simulink library "Computer_Library"  (Simulink 8.1)
settings: Solver=ode45  StartTime=0.0  StopTime=10.0  RelTol=1e-3
values from neighbouring files (symbols this model uses):
  A = 10    [CharTable.m]
  ARROW_DOWN = 48    [CharTable.m]
  ARROW_LEFT = 49    [CharTable.m]
  ARROW_RIGHT = 50    [CharTable.m]
  ARROW_UP = 47    [CharTable.m]
  ASTERISK = 39    [CharTable.m]
  B = 11    [CharTable.m]
  BACKSLASH = 43    [CharTable.m]
  C = 12    [CharTable.m]
  COLON = 40    [CharTable.m]
  COMMA = 53    [CharTable.m]
  CROSS = 38    [CharTable.m]
  CURSOR = 62    [CharTable.m]
  D = 13    [CharTable.m]
  DOT = 52    [CharTable.m]
  EQUAL = 44    [CharTable.m]
  EXCLAMATION_MARK = 55    [CharTable.m]
  F = 15    [CharTable.m]
  G = 16    [CharTable.m]
  GREATER_THAN = 46    [CharTable.m]
  H = 17    [CharTable.m]
  I = 18    [CharTable.m]
  J = 19    [CharTable.m]
  K = 20    [CharTable.m]
  L = 21    [CharTable.m]
  LEFT_PARENTHESES = 59    [CharTable.m]
  LESS_THAN = 45    [CharTable.m]
  M = 22    [CharTable.m]
  MINUS = 37    [CharTable.m]
  N = 23    [CharTable.m]
  O = 24    [CharTable.m]
  P = 25    [CharTable.m]
  PERCENT = 58    [CharTable.m]
  PLUS = 36    [CharTable.m]
  Q = 32    [CharTable.m]
  QUESTION_MARK = 54    [CharTable.m]
  QUOTE = 56    [CharTable.m]
  R = 26    [CharTable.m]
  RECTANGLE = 63    [CharTable.m]
  RIGHT_PARENTHESES = 60    [CharTable.m]
  RomCode = reshape(transpose(RomCode), [], 1)    [ROM.m]
  S = 27    [CharTable.m]
  SEMICOLON = 41    [CharTable.m]
  SHARP = 57    [CharTable.m]
  SLASH = 42    [CharTable.m]
  SPACE = 61    [CharTable.m]
  T = 28    [CharTable.m]
  U = 29    [CharTable.m]
  UNDERSCORE = 51    [CharTable.m]
  V = 30    [CharTable.m]
  W = 31    [CharTable.m]
  X = 33    [CharTable.m]
  Y = 34    [CharTable.m]
  Z = 35    [CharTable.m]
undefined symbols (not defined in the file or in its folder): char_0
libraries: Memory_Blocks_Lib x116, Byte_Multiplexers_Lib x44, commutil2 x18, Bit_Multiplexers_Lib x17, Decoders_Lib x9, simulink_extras x8, Logic_Operations_Lib x4, Byte_Demultiplexers_Lib x2, Arithmetic_Operations_Lib x2, dspsnks4 x1
(part 2 of 4)

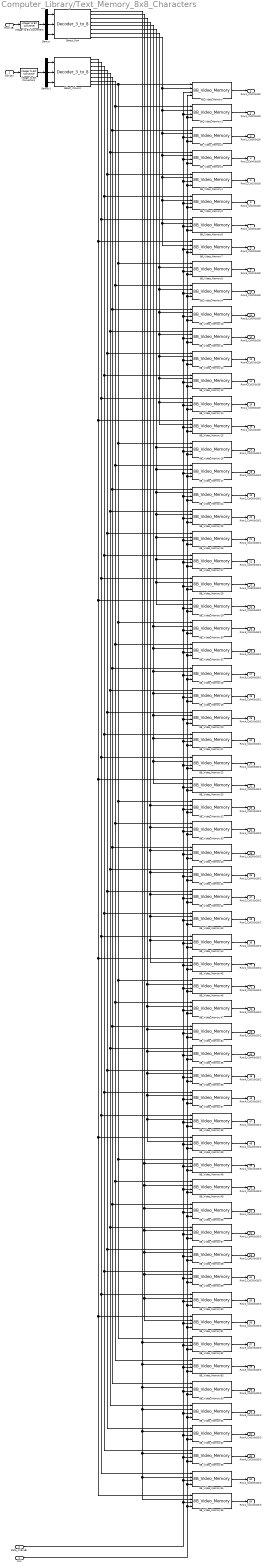
== system Computer_Library/Text_Memory_8x8_Characters ==
  Row(1B) : Inport
  Col(1B) : Inport  Port=2
  Data_In(8x1B) : Inport  Port=3
  CLK : Inport  Port=4
  8B_Video_Memory{,1..63} (64 alike) : Memory_Blocks_Lib/Memory_Blocks_Lib/8B_Video_Memory
  Demux : Demux  Outputs=3
  Demux1 : Demux  Outputs=3
  Integer to Bit Converter3 : commutil2/Integer to Bit Converter  nbits=3  signedInputValues=Unsigned  bitOrder=MSB first  outDtype=uint8
  Integer to Bit Converter4 : commutil2/Integer to Bit Converter  nbits=3  signedInputValues=Unsigned  bitOrder=MSB first  outDtype=uint8
  Select_Column : Decoders_Lib/Decoders_Lib/Decoder_3_to_8
  Select_Row : Decoders_Lib/Decoders_Lib/Decoder_3_to_8
  Row1_Col1(8x1B) : Outport
  Row1_Col2(8x1B) : Outport  Port=2
  Row1_Col3(8x1B) : Outport  Port=3
  Row1_Col4(8x1B) : Outport  Port=4
  Row2_Col1(8x1B) : Outport  Port=5
  Row2_Col2(8x1B) : Outport  Port=6
  Row2_Col3(8x1B) : Outport  Port=7
  Row2_Col4(8x1B) : Outport  Port=8
  Row3_Col1(8x1B) : Outport  Port=9
  Row3_Col2(8x1B) : Outport  Port=10
  Row3_Col3(8x1B) : Outport  Port=11
  Row3_Col4(8x1B) : Outport  Port=12
  Row4_Col1(8x1B) : Outport  Port=13
  Row4_Col2(8x1B) : Outport  Port=14
  Row4_Col3(8x1B) : Outport  Port=15
  Row4_Col4(8x1B) : Outport  Port=16
  Row1_Col1(8x1B)1 : Outport  Port=17
  Row1_Col2(8x1B)1 : Outport  Port=18
  Row1_Col3(8x1B)1 : Outport  Port=19
  Row1_Col4(8x1B)1 : Outport  Port=20
  Row2_Col1(8x1B)1 : Outport  Port=21
  Row2_Col2(8x1B)1 : Outport  Port=22
  Row2_Col3(8x1B)1 : Outport  Port=23
  Row2_Col4(8x1B)1 : Outport  Port=24
  Row3_Col1(8x1B)1 : Outport  Port=25
  Row3_Col2(8x1B)1 : Outport  Port=26
  Row3_Col3(8x1B)1 : Outport  Port=27
  Row3_Col4(8x1B)1 : Outport  Port=28
  Row4_Col1(8x1B)1 : Outport  Port=29
  Row4_Col2(8x1B)1 : Outport  Port=30
  Row4_Col3(8x1B)1 : Outport  Port=31
  Row4_Col4(8x1B)1 : Outport  Port=32
  Row1_Col1(8x1B)2 : Outport  Port=33
  Row1_Col2(8x1B)2 : Outport  Port=34
  Row1_Col3(8x1B)2 : Outport  Port=35
  Row1_Col4(8x1B)2 : Outport  Port=36
  Row2_Col1(8x1B)2 : Outport  Port=37
  Row2_Col2(8x1B)2 : Outport  Port=38
  Row2_Col3(8x1B)2 : Outport  Port=39
  Row2_Col4(8x1B)2 : Outport  Port=40
  Row3_Col1(8x1B)2 : Outport  Port=41
  Row3_Col2(8x1B)2 : Outport  Port=42
  Row3_Col3(8x1B)2 : Outport  Port=43
  Row3_Col4(8x1B)2 : Outport  Port=44
  Row4_Col1(8x1B)2 : Outport  Port=45
  Row4_Col2(8x1B)2 : Outport  Port=46
  Row4_Col3(8x1B)2 : Outport  Port=47
  Row4_Col4(8x1B)2 : Outport  Port=48
  Row1_Col1(8x1B)3 : Outport  Port=49
  Row1_Col2(8x1B)3 : Outport  Port=50
  Row1_Col3(8x1B)3 : Outport  Port=51
  Row1_Col4(8x1B)3 : Outport  Port=52
  Row2_Col1(8x1B)3 : Outport  Port=53
  Row2_Col2(8x1B)3 : Outport  Port=54
  Row2_Col3(8x1B)3 : Outport  Port=55
  Row2_Col4(8x1B)3 : Outport  Port=56
  Row3_Col1(8x1B)3 : Outport  Port=57
  Row3_Col2(8x1B)3 : Outport  Port=58
  Row3_Col3(8x1B)3 : Outport  Port=59
  Row3_Col4(8x1B)3 : Outport  Port=60
  Row4_Col1(8x1B)3 : Outport  Port=61
  Row4_Col2(8x1B)3 : Outport  Port=62
  Row4_Col3(8x1B)3 : Outport  Port=63
  Row4_Col4(8x1B)3 : Outport  Port=64
  wires:
  Row(1B)/1 -> Integer to Bit Converter3/1
  Integer to Bit Converter3/1 -> Demux/1
  Col(1B)/1 -> Integer to Bit Converter4/1
  Integer to Bit Converter4/1 -> Demux1/1
  8B_Video_Memory/1 -> Row1_Col1(8x1B)/1
  8B_Video_Memory1/1 -> Row1_Col2(8x1B)/1
  8B_Video_Memory2/1 -> Row1_Col3(8x1B)/1
  8B_Video_Memory3/1 -> Row1_Col4(8x1B)/1
  Select_Row/5 -> 8B_Video_Memory30/2, 8B_Video_Memory31/2, 8B_Video_Memory18/2, 8B_Video_Memory19/2, 8B_Video_Memory20/2, 8B_Video_Memory21/2, 8B_Video_Memory22/2, 8B_Video_Memory23/2
  Select_Row/6 -> 8B_Video_Memory16/2, 8B_Video_Memory17/2, 8B_Video_Memory24/2, 8B_Video_Memory25/2, 8B_Video_Memory26/2, 8B_Video_Memory27/2, 8B_Video_Memory28/2, 8B_Video_Memory29/2
  Select_Column/5 -> 8B_Video_Memory3/1, 8B_Video_Memory51/1, 8B_Video_Memory57/1, 8B_Video_Memory35/1, 8B_Video_Memory41/1, 8B_Video_Memory19/1, 8B_Video_Memory25/1, 8B_Video_Memory11/1
  Select_Column/6 -> 8B_Video_Memory2/1, 8B_Video_Memory50/1, 8B_Video_Memory56/1, 8B_Video_Memory34/1, 8B_Video_Memory40/1, 8B_Video_Memory18/1, 8B_Video_Memory24/1, 8B_Video_Memory10/1
  Select_Row/8 -> 8B_Video_Memory/2, 8B_Video_Memory1/2, 8B_Video_Memory2/2, 8B_Video_Memory3/2, 8B_Video_Memory4/2, 8B_Video_Memory5/2, 8B_Video_Memory6/2, 8B_Video_Memory7/2
  Select_Row/7 -> 8B_Video_Memory8/2, 8B_Video_Memory9/2, 8B_Video_Memory10/2, 8B_Video_Memory11/2, 8B_Video_Memory12/2, 8B_Video_Memory13/2, 8B_Video_Memory14/2, 8B_Video_Memory15/2
  Select_Column/8 -> 8B_Video_Memory/1, 8B_Video_Memory62/1, 8B_Video_Memory48/1, 8B_Video_Memory46/1, 8B_Video_Memory32/1, 8B_Video_Memory30/1, 8B_Video_Memory16/1, 8B_Video_Memory8/1
  Select_Column/7 -> 8B_Video_Memory1/1, 8B_Video_Memory63/1, 8B_Video_Memory49/1, 8B_Video_Memory47/1, 8B_Video_Memory33/1, 8B_Video_Memory31/1, 8B_Video_Memory17/1, 8B_Video_Memory9/1
  8B_Video_Memory4/1 -> Row2_Col1(8x1B)/1
  8B_Video_Memory5/1 -> Row2_Col2(8x1B)/1
  8B_Video_Memory6/1 -> Row2_Col3(8x1B)/1
  8B_Video_Memory7/1 -> Row2_Col4(8x1B)/1
  8B_Video_Memory8/1 -> Row3_Col1(8x1B)/1
  8B_Video_Memory9/1 -> Row3_Col2(8x1B)/1
  8B_Video_Memory10/1 -> Row3_Col3(8x1B)/1
  8B_Video_Memory11/1 -> Row3_Col4(8x1B)/1
  8B_Video_Memory12/1 -> Row4_Col1(8x1B)/1
  8B_Video_Memory13/1 -> Row4_Col2(8x1B)/1
  8B_Video_Memory14/1 -> Row4_Col3(8x1B)/1
  8B_Video_Memory15/1 -> Row4_Col4(8x1B)/1
  Demux/1 -> Select_Row/1
  Demux/2 -> Select_Row/2
  Demux1/1 -> Select_Column/1
  Demux1/2 -> Select_Column/2
  8B_Video_Memory16/1 -> Row1_Col1(8x1B)1/1
  8B_Video_Memory17/1 -> Row1_Col2(8x1B)1/1
  8B_Video_Memory24/1 -> Row1_Col3(8x1B)1/1
  8B_Video_Memory25/1 -> Row1_Col4(8x1B)1/1
  8B_Video_Memory26/1 -> Row2_Col1(8x1B)1/1
  8B_Video_Memory27/1 -> Row2_Col2(8x1B)1/1
  8B_Video_Memory28/1 -> Row2_Col3(8x1B)1/1
  8B_Video_Memory29/1 -> Row2_Col4(8x1B)1/1
  8B_Video_Memory30/1 -> Row3_Col1(8x1B)1/1
  8B_Video_Memory31/1 -> Row3_Col2(8x1B)1/1
  8B_Video_Memory18/1 -> Row3_Col3(8x1B)1/1
  8B_Video_Memory19/1 -> Row3_Col4(8x1B)1/1
  8B_Video_Memory20/1 -> Row4_Col1(8x1B)1/1
  8B_Video_Memory21/1 -> Row4_Col2(8x1B)1/1
  8B_Video_Memory22/1 -> Row4_Col3(8x1B)1/1
  8B_Video_Memory23/1 -> Row4_Col4(8x1B)1/1
  8B_Video_Memory32/1 -> Row1_Col1(8x1B)2/1
  8B_Video_Memory33/1 -> Row1_Col2(8x1B)2/1
  8B_Video_Memory40/1 -> Row1_Col3(8x1B)2/1
  8B_Video_Memory41/1 -> Row1_Col4(8x1B)2/1
  8B_Video_Memory42/1 -> Row2_Col1(8x1B)2/1
  8B_Video_Memory43/1 -> Row2_Col2(8x1B)2/1
  8B_Video_Memory44/1 -> Row2_Col3(8x1B)2/1
  8B_Video_Memory45/1 -> Row2_Col4(8x1B)2/1
  8B_Video_Memory46/1 -> Row3_Col1(8x1B)2/1
  8B_Video_Memory47/1 -> Row3_Col2(8x1B)2/1
  8B_Video_Memory34/1 -> Row3_Col3(8x1B)2/1
  8B_Video_Memory35/1 -> Row3_Col4(8x1B)2/1
  8B_Video_Memory36/1 -> Row4_Col1(8x1B)2/1
  8B_Video_Memory37/1 -> Row4_Col2(8x1B)2/1
  8B_Video_Memory38/1 -> Row4_Col3(8x1B)2/1
  8B_Video_Memory39/1 -> Row4_Col4(8x1B)2/1
  8B_Video_Memory48/1 -> Row1_Col1(8x1B)3/1
  8B_Video_Memory49/1 -> Row1_Col2(8x1B)3/1
  8B_Video_Memory56/1 -> Row1_Col3(8x1B)3/1
  8B_Video_Memory57/1 -> Row1_Col4(8x1B)3/1
  8B_Video_Memory58/1 -> Row2_Col1(8x1B)3/1
  8B_Video_Memory59/1 -> Row2_Col2(8x1B)3/1
  8B_Video_Memory60/1 -> Row2_Col3(8x1B)3/1
  8B_Video_Memory61/1 -> Row2_Col4(8x1B)3/1
  8B_Video_Memory62/1 -> Row3_Col1(8x1B)3/1
  8B_Video_Memory63/1 -> Row3_Col2(8x1B)3/1
  8B_Video_Memory50/1 -> Row3_Col3(8x1B)3/1
  8B_Video_Memory51/1 -> Row3_Col4(8x1B)3/1
  8B_Video_Memory52/1 -> Row4_Col1(8x1B)3/1
  8B_Video_Memory53/1 -> Row4_Col2(8x1B)3/1
  8B_Video_Memory54/1 -> Row4_Col3(8x1B)3/1
  8B_Video_Memory55/1 -> Row4_Col4(8x1B)3/1
  Data_In(8x1B)/1 -> 8B_Video_Memory55/3, 8B_Video_Memory54/3, 8B_Video_Memory53/3, 8B_Video_Memory52/3, 8B_Video_Memory51/3, 8B_Video_Memory50/3, 8B_Video_Memory63/3, 8B_Video_Memory62/3, 8B_Video_Memory61/3, 8B_Video_Memory60/3, 8B_Video_Memory59/3, 8B_Video_Memory58/3, 8B_Video_Memory57/3, 8B_Video_Memory56/3, 8B_Video_Memory49/3, 8B_Video_Memory48/3, 8B_Video_Memory39/3, 8B_Video_Memory38/3, 8B_Video_Memory37/3, 8B_Video_Memory36/3, 8B_Video_Memory35/3, 8B_Video_Memory34/3, 8B_Video_Memory47/3, 8B_Video_Memory46/3, 8B_Video_Memory45/3, 8B_Video_Memory44/3, 8B_Video_Memory43/3, 8B_Video_Memory42/3, 8B_Video_Memory41/3, 8B_Video_Memory40/3, 8B_Video_Memory33/3, 8B_Video_Memory32/3, 8B_Video_Memory23/3, 8B_Video_Memory22/3, 8B_Video_Memory21/3, 8B_Video_Memory20/3, 8B_Video_Memory19/3, 8B_Video_Memory18/3, 8B_Video_Memory31/3, 8B_Video_Memory30/3, 8B_Video_Memory29/3, 8B_Video_Memory28/3, 8B_Video_Memory27/3, 8B_Video_Memory26/3, 8B_Video_Memory25/3, 8B_Video_Memory24/3, 8B_Video_Memory17/3, 8B_Video_Memory16/3, 8B_Video_Memory15/3, 8B_Video_Memory14/3, 8B_Video_Memory13/3, 8B_Video_Memory12/3, 8B_Video_Memory11/3, 8B_Video_Memory10/3, 8B_Video_Memory9/3, 8B_Video_Memory8/3, 8B_Video_Memory6/3, 8B_Video_Memory5/3, 8B_Video_Memory4/3, 8B_Video_Memory2/3, 8B_Video_Memory1/3, 8B_Video_Memory/3, 8B_Video_Memory3/3, 8B_Video_Memory7/3
  CLK/1 -> 8B_Video_Memory55/4, 8B_Video_Memory54/4, 8B_Video_Memory53/4, 8B_Video_Memory52/4, 8B_Video_Memory51/4, 8B_Video_Memory50/4, 8B_Video_Memory63/4, 8B_Video_Memory62/4, 8B_Video_Memory61/4, 8B_Video_Memory60/4, 8B_Video_Memory59/4, 8B_Video_Memory58/4, 8B_Video_Memory57/4, 8B_Video_Memory56/4, 8B_Video_Memory49/4, 8B_Video_Memory48/4, 8B_Video_Memory39/4, 8B_Video_Memory38/4, 8B_Video_Memory37/4, 8B_Video_Memory36/4, 8B_Video_Memory35/4, 8B_Video_Memory34/4, 8B_Video_Memory47/4, 8B_Video_Memory46/4, 8B_Video_Memory45/4, 8B_Video_Memory44/4, 8B_Video_Memory43/4, 8B_Video_Memory42/4, 8B_Video_Memory41/4, 8B_Video_Memory40/4, 8B_Video_Memory33/4, 8B_Video_Memory32/4, 8B_Video_Memory23/4, 8B_Video_Memory22/4, 8B_Video_Memory21/4, 8B_Video_Memory20/4, 8B_Video_Memory19/4, 8B_Video_Memory18/4, 8B_Video_Memory31/4, 8B_Video_Memory30/4, 8B_Video_Memory29/4, 8B_Video_Memory28/4, 8B_Video_Memory27/4, 8B_Video_Memory26/4, 8B_Video_Memory25/4, 8B_Video_Memory24/4, 8B_Video_Memory17/4, 8B_Video_Memory16/4, 8B_Video_Memory15/4, 8B_Video_Memory14/4, 8B_Video_Memory13/4, 8B_Video_Memory12/4, 8B_Video_Memory11/4, 8B_Video_Memory10/4, 8B_Video_Memory9/4, 8B_Video_Memory8/4, 8B_Video_Memory7/4, 8B_Video_Memory6/4, 8B_Video_Memory5/4, 8B_Video_Memory4/4, 8B_Video_Memory3/4, 8B_Video_Memory2/4, 8B_Video_Memory1/4, 8B_Video_Memory/4
  Select_Row/4 -> 8B_Video_Memory32/2, 8B_Video_Memory33/2, 8B_Video_Memory40/2, 8B_Video_Memory41/2, 8B_Video_Memory42/2, 8B_Video_Memory43/2, 8B_Video_Memory44/2, 8B_Video_Memory45/2
  Select_Row/3 -> 8B_Video_Memory46/2, 8B_Video_Memory47/2, 8B_Video_Memory34/2, 8B_Video_Memory35/2, 8B_Video_Memory36/2, 8B_Video_Memory37/2, 8B_Video_Memory38/2, 8B_Video_Memory39/2
  Select_Row/2 -> 8B_Video_Memory48/2, 8B_Video_Memory49/2, 8B_Video_Memory56/2, 8B_Video_Memory57/2, 8B_Video_Memory58/2, 8B_Video_Memory60/2, 8B_Video_Memory61/2, 8B_Video_Memory59/2
  Select_Row/1 -> 8B_Video_Memory62/2, 8B_Video_Memory63/2, 8B_Video_Memory50/2, 8B_Video_Memory51/2, 8B_Video_Memory52/2, 8B_Video_Memory53/2, 8B_Video_Memory54/2, 8B_Video_Memory55/2
  Select_Column/4 -> 8B_Video_Memory52/1, 8B_Video_Memory58/1, 8B_Video_Memory36/1, 8B_Video_Memory42/1, 8B_Video_Memory20/1, 8B_Video_Memory26/1, 8B_Video_Memory12/1, 8B_Video_Memory4/1
  Select_Column/3 -> 8B_Video_Memory53/1, 8B_Video_Memory59/1, 8B_Video_Memory37/1, 8B_Video_Memory43/1, 8B_Video_Memory21/1, 8B_Video_Memory27/1, 8B_Video_Memory13/1, 8B_Video_Memory5/1
  Select_Column/2 -> 8B_Video_Memory54/1, 8B_Video_Memory60/1, 8B_Video_Memory38/1, 8B_Video_Memory44/1, 8B_Video_Memory22/1, 8B_Video_Memory28/1, 8B_Video_Memory14/1, 8B_Video_Memory6/1
  Select_Column/1 -> 8B_Video_Memory55/1, 8B_Video_Memory61/1, 8B_Video_Memory39/1, 8B_Video_Memory45/1, 8B_Video_Memory23/1, 8B_Video_Memory29/1, 8B_Video_Memory15/1, 8B_Video_Memory7/1
  Demux/3 -> Select_Row/3
  Demux1/3 -> Select_Column/3

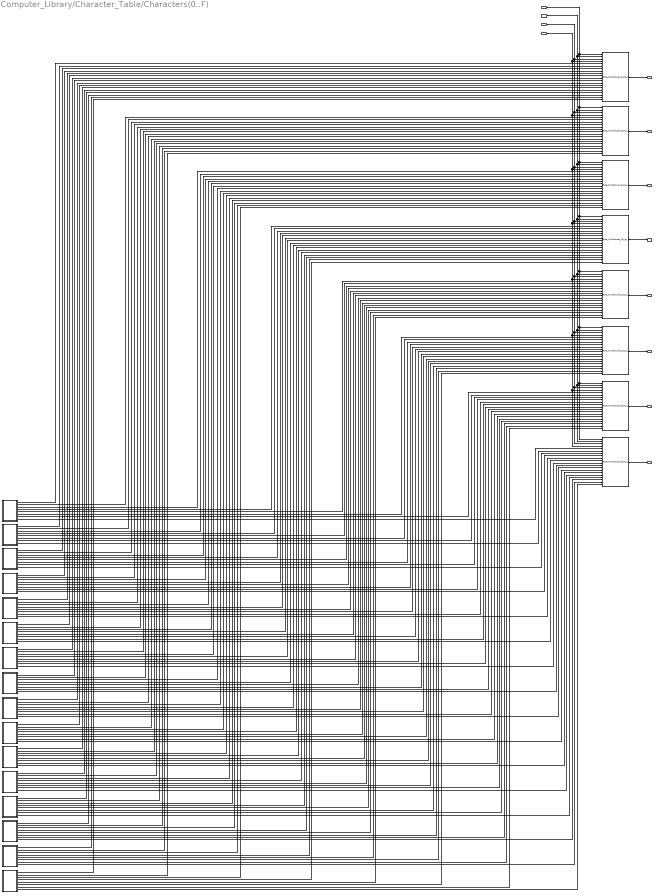
== system Computer_Library/Character_Table/Characters(0..F) ==
  Address_3_In(1b) : Inport
  Address_2_In(1b) : Inport  Port=2
  Address_1_In(1b) : Inport  Port=3
  Address_0_In(1b) : Inport  Port=4
  16_to_1_Byte_Multiplexer{,1..7} (8 alike) : Byte_Multiplexers_Lib/Byte_Multiplexers_Lib/Byte_Multiplexer_16_to_1
  Char_0 : Subsystem
  Char_1 : Subsystem
  Char_2 : Subsystem
  Char_3 : Subsystem
  Char_4 : Subsystem
  Char_5 : Subsystem
  Char_6 : Subsystem
  Char_7 : Subsystem
  Char_8 : Subsystem
  Char_9 : Subsystem
  Char_A : Subsystem
  Char_B : Subsystem
  Char_C : Subsystem
  Char_D : Subsystem
  Char_E : Subsystem
  Char_F : Subsystem
  Column_1(1B) : Outport
  Column_2(1B) : Outport  Port=2
  Column_3(1B) : Outport  Port=3
  Column_4(1B) : Outport  Port=4
  Column_5(1B) : Outport  Port=5
  Column_6(1B) : Outport  Port=6
  Column_7(1B) : Outport  Port=7
  Column_8(1B) : Outport  Port=8
  wires:
  Char_F/1(Column_1(1B)) -> 16_to_1_Byte_Multiplexer/5
  Char_E/1(Column_1(1B)) -> 16_to_1_Byte_Multiplexer/6
  Char_D/1(Column_1(1B)) -> 16_to_1_Byte_Multiplexer/7
  Char_C/1(Column_1(1B)) -> 16_to_1_Byte_Multiplexer/8
  Char_B/1(Column_1(1B)) -> 16_to_1_Byte_Multiplexer/9
  Char_A/1(Column_1(1B)) -> 16_to_1_Byte_Multiplexer/10
  Char_9/1(Column_1(1B)) -> 16_to_1_Byte_Multiplexer/11
  Char_8/1(Column_1(1B)) -> 16_to_1_Byte_Multiplexer/12
  Char_7/1(Column_1(1B)) -> 16_to_1_Byte_Multiplexer/13
  Char_6/1(Column_1(1B)) -> 16_to_1_Byte_Multiplexer/14
  Char_5/1(Column_1(1B)) -> 16_to_1_Byte_Multiplexer/15
  Char_4/1(Column_1(1B)) -> 16_to_1_Byte_Multiplexer/16
  Char_3/1(Column_1(1B)) -> 16_to_1_Byte_Multiplexer/17
  Char_2/1(Column_1(1B)) -> 16_to_1_Byte_Multiplexer/18
  Char_1/1(Column_1(1B)) -> 16_to_1_Byte_Multiplexer/19
  Char_0/1(Column_1(1B)) -> 16_to_1_Byte_Multiplexer/20
  Char_F/2(Column_2(1B)) -> 16_to_1_Byte_Multiplexer1/5
  Char_0/2(Column_2(1B)) -> 16_to_1_Byte_Multiplexer1/20
  Char_1/2(Column_2(1B)) -> 16_to_1_Byte_Multiplexer1/19
  Char_2/2(Column_2(1B)) -> 16_to_1_Byte_Multiplexer1/18
  Char_3/2(Column_2(1B)) -> 16_to_1_Byte_Multiplexer1/17
  Char_4/2(Column_2(1B)) -> 16_to_1_Byte_Multiplexer1/16
  Char_5/2(Column_2(1B)) -> 16_to_1_Byte_Multiplexer1/15
  Char_6/2(Column_2(1B)) -> 16_to_1_Byte_Multiplexer1/14
  Char_7/2(Column_2(1B)) -> 16_to_1_Byte_Multiplexer1/13
  Char_8/2(Column_2(1B)) -> 16_to_1_Byte_Multiplexer1/12
  Char_9/2(Column_2(1B)) -> 16_to_1_Byte_Multiplexer1/11
  Char_A/2(Column_2(1B)) -> 16_to_1_Byte_Multiplexer1/10
  Char_B/2(Column_2(1B)) -> 16_to_1_Byte_Multiplexer1/9
  Char_C/2(Column_2(1B)) -> 16_to_1_Byte_Multiplexer1/8
  Char_D/2(Column_2(1B)) -> 16_to_1_Byte_Multiplexer1/7
  Char_E/2(Column_2(1B)) -> 16_to_1_Byte_Multiplexer1/6
  Char_0/3(Column_3(1B)) -> 16_to_1_Byte_Multiplexer2/20
  Char_1/3(Column_3(1B)) -> 16_to_1_Byte_Multiplexer2/19
  Char_2/3(Column_3(1B)) -> 16_to_1_Byte_Multiplexer2/18
  Char_3/3(Column_3(1B)) -> 16_to_1_Byte_Multiplexer2/17
  Char_4/3(Column_3(1B)) -> 16_to_1_Byte_Multiplexer2/16
  Char_5/3(Column_3(1B)) -> 16_to_1_Byte_Multiplexer2/15
  Char_6/3(Column_3(1B)) -> 16_to_1_Byte_Multiplexer2/14
  Char_7/3(Column_3(1B)) -> 16_to_1_Byte_Multiplexer2/13
  Char_8/3(Column_3(1B)) -> 16_to_1_Byte_Multiplexer2/12
  Char_9/3(Column_3(1B)) -> 16_to_1_Byte_Multiplexer2/11
  Char_A/3(Column_3(1B)) -> 16_to_1_Byte_Multiplexer2/10
  Char_B/3(Column_3(1B)) -> 16_to_1_Byte_Multiplexer2/9
  Char_C/3(Column_3(1B)) -> 16_to_1_Byte_Multiplexer2/8
  Char_D/3(Column_3(1B)) -> 16_to_1_Byte_Multiplexer2/7
  Char_E/3(Column_3(1B)) -> 16_to_1_Byte_Multiplexer2/6
  Char_F/3(Column_3(1B)) -> 16_to_1_Byte_Multiplexer2/5
  Char_0/4(Column_4(1B)) -> 16_to_1_Byte_Multiplexer3/20
  Char_1/4(Column_4(1B)) -> 16_to_1_Byte_Multiplexer3/19
  Char_2/4(Column_4(1B)) -> 16_to_1_Byte_Multiplexer3/18
  Char_3/4(Column_4(1B)) -> 16_to_1_Byte_Multiplexer3/17
  Char_4/4(Column_4(1B)) -> 16_to_1_Byte_Multiplexer3/16
  Char_5/4(Column_4(1B)) -> 16_to_1_Byte_Multiplexer3/15
  Char_6/4(Column_4(1B)) -> 16_to_1_Byte_Multiplexer3/14
  Char_7/4(Column_4(1B)) -> 16_to_1_Byte_Multiplexer3/13
  Char_8/4(Column_4(1B)) -> 16_to_1_Byte_Multiplexer3/12
  Char_9/4(Column_4(1B)) -> 16_to_1_Byte_Multiplexer3/11
  Char_A/4(Column_4(1B)) -> 16_to_1_Byte_Multiplexer3/10
  Char_B/4(Column_4(1B)) -> 16_to_1_Byte_Multiplexer3/9
  Char_C/4(Column_4(1B)) -> 16_to_1_Byte_Multiplexer3/8
  Char_D/4(Column_4(1B)) -> 16_to_1_Byte_Multiplexer3/7
  Char_E/4(Column_4(1B)) -> 16_to_1_Byte_Multiplexer3/6
  Char_F/4(Column_4(1B)) -> 16_to_1_Byte_Multiplexer3/5
  Char_0/5(Column_5(1B)) -> 16_to_1_Byte_Multiplexer4/20
  Char_1/5(Column_5(1B)) -> 16_to_1_Byte_Multiplexer4/19
  Char_2/5(Column_5(1B)) -> 16_to_1_Byte_Multiplexer4/18
  Char_3/5(Column_5(1B)) -> 16_to_1_Byte_Multiplexer4/17
  Char_4/5(Column_5(1B)) -> 16_to_1_Byte_Multiplexer4/16
  Char_5/5(Column_5(1B)) -> 16_to_1_Byte_Multiplexer4/15
  Char_7/5(Column_5(1B)) -> 16_to_1_Byte_Multiplexer4/13
  Char_6/5(Column_5(1B)) -> 16_to_1_Byte_Multiplexer4/14
  Char_8/5(Column_5(1B)) -> 16_to_1_Byte_Multiplexer4/12
  Char_9/5(Column_5(1B)) -> 16_to_1_Byte_Multiplexer4/11
  Char_A/5(Column_5(1B)) -> 16_to_1_Byte_Multiplexer4/10
  Char_B/5(Column_5(1B)) -> 16_to_1_Byte_Multiplexer4/9
  Char_C/5(Column_5(1B)) -> 16_to_1_Byte_Multiplexer4/8
  Char_D/5(Column_5(1B)) -> 16_to_1_Byte_Multiplexer4/7
  Char_E/5(Column_5(1B)) -> 16_to_1_Byte_Multiplexer4/6
  Char_F/5(Column_5(1B)) -> 16_to_1_Byte_Multiplexer4/5
  Char_0/6(Column_6(1B)) -> 16_to_1_Byte_Multiplexer5/20
  Char_1/6(Column_6(1B)) -> 16_to_1_Byte_Multiplexer5/19
  Char_2/6(Column_6(1B)) -> 16_to_1_Byte_Multiplexer5/18
  Char_3/6(Column_6(1B)) -> 16_to_1_Byte_Multiplexer5/17
  Char_4/6(Column_6(1B)) -> 16_to_1_Byte_Multiplexer5/16
  Char_5/6(Column_6(1B)) -> 16_to_1_Byte_Multiplexer5/15
  Char_6/6(Column_6(1B)) -> 16_to_1_Byte_Multiplexer5/14
  Char_7/6(Column_6(1B)) -> 16_to_1_Byte_Multiplexer5/13
  Char_8/6(Column_6(1B)) -> 16_to_1_Byte_Multiplexer5/12
  Char_9/6(Column_6(1B)) -> 16_to_1_Byte_Multiplexer5/11
  Char_A/6(Column_6(1B)) -> 16_to_1_Byte_Multiplexer5/10
  Char_B/6(Column_6(1B)) -> 16_to_1_Byte_Multiplexer5/9
  Char_C/7(Column_7(1B)) -> 16_to_1_Byte_Multiplexer6/8
  Char_C/6(Column_6(1B)) -> 16_to_1_Byte_Multiplexer5/8
  Char_D/6(Column_6(1B)) -> 16_to_1_Byte_Multiplexer5/7
  Char_E/6(Column_6(1B)) -> 16_to_1_Byte_Multiplexer5/6
  Char_F/6(Column_6(1B)) -> 16_to_1_Byte_Multiplexer5/5
  Char_0/7(Column_7(1B)) -> 16_to_1_Byte_Multiplexer6/20
  Char_1/7(Column_7(1B)) -> 16_to_1_Byte_Multiplexer6/19
  Char_2/7(Column_7(1B)) -> 16_to_1_Byte_Multiplexer6/18
  Char_3/7(Column_7(1B)) -> 16_to_1_Byte_Multiplexer6/17
  Char_4/7(Column_7(1B)) -> 16_to_1_Byte_Multiplexer6/16
  Char_5/7(Column_7(1B)) -> 16_to_1_Byte_Multiplexer6/15
  Char_6/7(Column_7(1B)) -> 16_to_1_Byte_Multiplexer6/14
  Char_7/7(Column_7(1B)) -> 16_to_1_Byte_Multiplexer6/13
  Char_8/7(Column_7(1B)) -> 16_to_1_Byte_Multiplexer6/12
  Char_9/7(Column_7(1B)) -> 16_to_1_Byte_Multiplexer6/11
  Char_A/7(Column_7(1B)) -> 16_to_1_Byte_Multiplexer6/10
  Char_B/7(Column_7(1B)) -> 16_to_1_Byte_Multiplexer6/9
  Char_D/7(Column_7(1B)) -> 16_to_1_Byte_Multiplexer6/7
  Char_E/7(Column_7(1B)) -> 16_to_1_Byte_Multiplexer6/6
  Char_F/7(Column_7(1B)) -> 16_to_1_Byte_Multiplexer6/5
  Char_0/8(Column_8(1B)) -> 16_to_1_Byte_Multiplexer7/20
  Char_1/8(Column_8(1B)) -> 16_to_1_Byte_Multiplexer7/19
  Char_2/8(Column_8(1B)) -> 16_to_1_Byte_Multiplexer7/18
  Char_3/8(Column_8(1B)) -> 16_to_1_Byte_Multiplexer7/17
  Char_4/8(Column_8(1B)) -> 16_to_1_Byte_Multiplexer7/16
  Char_5/8(Column_8(1B)) -> 16_to_1_Byte_Multiplexer7/15
  Char_6/8(Column_8(1B)) -> 16_to_1_Byte_Multiplexer7/14
  Char_7/8(Column_8(1B)) -> 16_to_1_Byte_Multiplexer7/13
  Char_8/8(Column_8(1B)) -> 16_to_1_Byte_Multiplexer7/12
  Char_9/8(Column_8(1B)) -> 16_to_1_Byte_Multiplexer7/11
  Char_A/8(Column_8(1B)) -> 16_to_1_Byte_Multiplexer7/10
  Char_B/8(Column_8(1B)) -> 16_to_1_Byte_Multiplexer7/9
  Char_C/8(Column_8(1B)) -> 16_to_1_Byte_Multiplexer7/8
  Char_D/8(Column_8(1B)) -> 16_to_1_Byte_Multiplexer7/7
  Char_E/8(Column_8(1B)) -> 16_to_1_Byte_Multiplexer7/6
  Char_F/8(Column_8(1B)) -> 16_to_1_Byte_Multiplexer7/5
  16_to_1_Byte_Multiplexer/1 -> Column_1(1B)/1
  16_to_1_Byte_Multiplexer1/1 -> Column_2(1B)/1
  16_to_1_Byte_Multiplexer2/1 -> Column_3(1B)/1
  16_to_1_Byte_Multiplexer3/1 -> Column_4(1B)/1
  16_to_1_Byte_Multiplexer4/1 -> Column_5(1B)/1
  16_to_1_Byte_Multiplexer5/1 -> Column_6(1B)/1
  16_to_1_Byte_Multiplexer6/1 -> Column_7(1B)/1
  16_to_1_Byte_Multiplexer7/1 -> Column_8(1B)/1
  Address_0_In(1b)/1 -> 16_to_1_Byte_Multiplexer/4, 16_to_1_Byte_Multiplexer1/4, 16_to_1_Byte_Multiplexer2/4, 16_to_1_Byte_Multiplexer3/4, 16_to_1_Byte_Multiplexer4/4, 16_to_1_Byte_Multiplexer5/4, 16_to_1_Byte_Multiplexer6/4, 16_to_1_Byte_Multiplexer7/4
  Address_1_In(1b)/1 -> 16_to_1_Byte_Multiplexer/3, 16_to_1_Byte_Multiplexer1/3, 16_to_1_Byte_Multiplexer2/3, 16_to_1_Byte_Multiplexer3/3, 16_to_1_Byte_Multiplexer4/3, 16_to_1_Byte_Multiplexer5/3, 16_to_1_Byte_Multiplexer6/3, 16_to_1_Byte_Multiplexer7/3
  Address_2_In(1b)/1 -> 16_to_1_Byte_Multiplexer/2, 16_to_1_Byte_Multiplexer1/2, 16_to_1_Byte_Multiplexer2/2, 16_to_1_Byte_Multiplexer3/2, 16_to_1_Byte_Multiplexer4/2, 16_to_1_Byte_Multiplexer5/2, 16_to_1_Byte_Multiplexer6/2, 16_to_1_Byte_Multiplexer7/2
  Address_3_In(1b)/1 -> 16_to_1_Byte_Multiplexer/1, 16_to_1_Byte_Multiplexer1/1, 16_to_1_Byte_Multiplexer2/1, 16_to_1_Byte_Multiplexer3/1, 16_to_1_Byte_Multiplexer4/1, 16_to_1_Byte_Multiplexer5/1, 16_to_1_Byte_Multiplexer6/1, 16_to_1_Byte_Multiplexer7/1

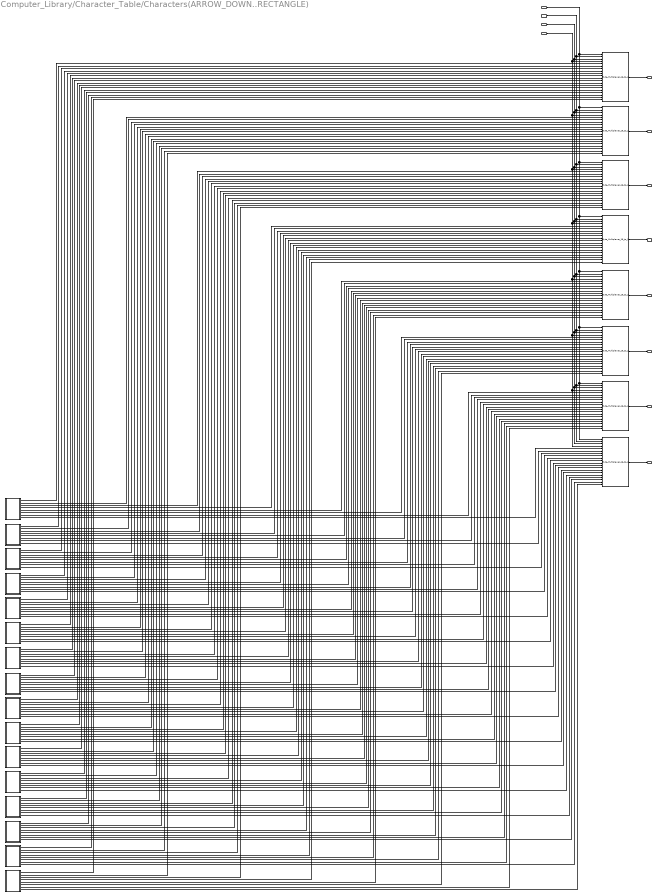
== system Computer_Library/Character_Table/Characters(ARROW_DOWN..RECTANGLE) ==
  Address_3_In(1b) : Inport
  Address_2_In(1b) : Inport  Port=2
  Address_1_In(1b) : Inport  Port=3
  Address_0_In(1b) : Inport  Port=4
  16_to_1_Byte_Multiplexer{,1..7} (8 alike) : Byte_Multiplexers_Lib/Byte_Multiplexers_Lib/Byte_Multiplexer_16_to_1
  Char_ARROW_DOWN : Subsystem
  Char_ARROW_LEFT : Subsystem
  Char_ARROW_RIGHT : Subsystem
  Char_COMMA : Subsystem
  Char_CURSOR : Subsystem
  Char_DOT : Subsystem
  Char_EXCLAMATION_MARK : Subsystem
  Char_LEFT_PARENTHESES : Subsystem
  Char_PERCENT : Subsystem
  Char_QUESTION_MARK : Subsystem
  Char_QUOTE : Subsystem
  Char_RECTANGLE : Subsystem
  Char_RIGHT_PARENTHESES : Subsystem
  Char_SHARP : Subsystem
  Char_SPACE : Subsystem
  Char_UNDERSCORE : Subsystem
  Column_1(1B) : Outport
  Column_2(1B) : Outport  Port=2
  Column_3(1B) : Outport  Port=3
  Column_4(1B) : Outport  Port=4
  Column_5(1B) : Outport  Port=5
  Column_6(1B) : Outport  Port=6
  Column_7(1B) : Outport  Port=7
  Column_8(1B) : Outport  Port=8
  wires:
  Char_RECTANGLE/1(Column_1(1B)) -> 16_to_1_Byte_Multiplexer/5
  Char_CURSOR/1(Column_1(1B)) -> 16_to_1_Byte_Multiplexer/6
  Char_SPACE/1(Column_1(1B)) -> 16_to_1_Byte_Multiplexer/7
  Char_RIGHT_PARENTHESES/1(Column_1(1B)) -> 16_to_1_Byte_Multiplexer/8
  Char_LEFT_PARENTHESES/1(Column_1(1B)) -> 16_to_1_Byte_Multiplexer/9
  Char_PERCENT/1(Column_1(1B)) -> 16_to_1_Byte_Multiplexer/10
  Char_SHARP/1(Column_1(1B)) -> 16_to_1_Byte_Multiplexer/11
  Char_QUOTE/1(Column_1(1B)) -> 16_to_1_Byte_Multiplexer/12
  Char_EXCLAMATION_MARK/1(Column_1(1B)) -> 16_to_1_Byte_Multiplexer/13
  Char_QUESTION_MARK/1(Column_1(1B)) -> 16_to_1_Byte_Multiplexer/14
  Char_COMMA/1(Column_1(1B)) -> 16_to_1_Byte_Multiplexer/15
  Char_DOT/1(Column_1(1B)) -> 16_to_1_Byte_Multiplexer/16
  Char_UNDERSCORE/1(Column_1(1B)) -> 16_to_1_Byte_Multiplexer/17
  Char_ARROW_RIGHT/1(Column_1(1B)) -> 16_to_1_Byte_Multiplexer/18
  Char_ARROW_LEFT/1(Column_1(1B)) -> 16_to_1_Byte_Multiplexer/19
  Char_ARROW_DOWN/1(Column_1(1B)) -> 16_to_1_Byte_Multiplexer/20
  Char_RECTANGLE/2(Column_2(1B)) -> 16_to_1_Byte_Multiplexer1/5
  Char_ARROW_DOWN/2(Column_2(1B)) -> 16_to_1_Byte_Multiplexer1/20
  Char_ARROW_LEFT/2(Column_2(1B)) -> 16_to_1_Byte_Multiplexer1/19
  Char_ARROW_RIGHT/2(Column_2(1B)) -> 16_to_1_Byte_Multiplexer1/18
  Char_UNDERSCORE/2(Column_2(1B)) -> 16_to_1_Byte_Multiplexer1/17
  Char_DOT/2(Column_2(1B)) -> 16_to_1_Byte_Multiplexer1/16
  Char_COMMA/2(Column_2(1B)) -> 16_to_1_Byte_Multiplexer1/15
  Char_QUESTION_MARK/2(Column_2(1B)) -> 16_to_1_Byte_Multiplexer1/14
  Char_EXCLAMATION_MARK/2(Column_2(1B)) -> 16_to_1_Byte_Multiplexer1/13
  Char_QUOTE/2(Column_2(1B)) -> 16_to_1_Byte_Multiplexer1/12
  Char_SHARP/2(Column_2(1B)) -> 16_to_1_Byte_Multiplexer1/11
  Char_PERCENT/2(Column_2(1B)) -> 16_to_1_Byte_Multiplexer1/10
  Char_LEFT_PARENTHESES/2(Column_2(1B)) -> 16_to_1_Byte_Multiplexer1/9
  Char_RIGHT_PARENTHESES/2(Column_2(1B)) -> 16_to_1_Byte_Multiplexer1/8
  Char_SPACE/2(Column_2(1B)) -> 16_to_1_Byte_Multiplexer1/7
  Char_CURSOR/2(Column_2(1B)) -> 16_to_1_Byte_Multiplexer1/6
  Char_ARROW_DOWN/3(Column_3(1B)) -> 16_to_1_Byte_Multiplexer2/20
  Char_ARROW_LEFT/3(Column_3(1B)) -> 16_to_1_Byte_Multiplexer2/19
  Char_ARROW_RIGHT/3(Column_3(1B)) -> 16_to_1_Byte_Multiplexer2/18
  Char_UNDERSCORE/3(Column_3(1B)) -> 16_to_1_Byte_Multiplexer2/17
  Char_DOT/3(Column_3(1B)) -> 16_to_1_Byte_Multiplexer2/16
  Char_COMMA/3(Column_3(1B)) -> 16_to_1_Byte_Multiplexer2/15
  Char_QUESTION_MARK/3(Column_3(1B)) -> 16_to_1_Byte_Multiplexer2/14
  Char_EXCLAMATION_MARK/3(Column_3(1B)) -> 16_to_1_Byte_Multiplexer2/13
  Char_QUOTE/3(Column_3(1B)) -> 16_to_1_Byte_Multiplexer2/12
  Char_SHARP/3(Column_3(1B)) -> 16_to_1_Byte_Multiplexer2/11
  Char_PERCENT/3(Column_3(1B)) -> 16_to_1_Byte_Multiplexer2/10
  Char_LEFT_PARENTHESES/3(Column_3(1B)) -> 16_to_1_Byte_Multiplexer2/9
  Char_RIGHT_PARENTHESES/3(Column_3(1B)) -> 16_to_1_Byte_Multiplexer2/8
  Char_SPACE/3(Column_3(1B)) -> 16_to_1_Byte_Multiplexer2/7
  Char_CURSOR/3(Column_3(1B)) -> 16_to_1_Byte_Multiplexer2/6
  Char_RECTANGLE/3(Column_3(1B)) -> 16_to_1_Byte_Multiplexer2/5
  Char_ARROW_DOWN/4(Column_4(1B)) -> 16_to_1_Byte_Multiplexer3/20
  Char_ARROW_LEFT/4(Column_4(1B)) -> 16_to_1_Byte_Multiplexer3/19
  Char_ARROW_RIGHT/4(Column_4(1B)) -> 16_to_1_Byte_Multiplexer3/18
  Char_UNDERSCORE/4(Column_4(1B)) -> 16_to_1_Byte_Multiplexer3/17
  Char_DOT/4(Column_4(1B)) -> 16_to_1_Byte_Multiplexer3/16
  Char_COMMA/4(Column_4(1B)) -> 16_to_1_Byte_Multiplexer3/15
  Char_QUESTION_MARK/4(Column_4(1B)) -> 16_to_1_Byte_Multiplexer3/14
  Char_EXCLAMATION_MARK/4(Column_4(1B)) -> 16_to_1_Byte_Multiplexer3/13
  Char_QUOTE/4(Column_4(1B)) -> 16_to_1_Byte_Multiplexer3/12
  Char_SHARP/4(Column_4(1B)) -> 16_to_1_Byte_Multiplexer3/11
  Char_PERCENT/4(Column_4(1B)) -> 16_to_1_Byte_Multiplexer3/10
  Char_LEFT_PARENTHESES/4(Column_4(1B)) -> 16_to_1_Byte_Multiplexer3/9
  Char_RIGHT_PARENTHESES/4(Column_4(1B)) -> 16_to_1_Byte_Multiplexer3/8
  Char_SPACE/4(Column_4(1B)) -> 16_to_1_Byte_Multiplexer3/7
  Char_CURSOR/4(Column_4(1B)) -> 16_to_1_Byte_Multiplexer3/6
  Char_RECTANGLE/4(Column_4(1B)) -> 16_to_1_Byte_Multiplexer3/5
  Char_ARROW_DOWN/5(Column_5(1B)) -> 16_to_1_Byte_Multiplexer4/20
  Char_ARROW_LEFT/5(Column_5(1B)) -> 16_to_1_Byte_Multiplexer4/19
  Char_ARROW_RIGHT/5(Column_5(1B)) -> 16_to_1_Byte_Multiplexer4/18
  Char_UNDERSCORE/5(Column_5(1B)) -> 16_to_1_Byte_Multiplexer4/17
  Char_DOT/5(Column_5(1B)) -> 16_to_1_Byte_Multiplexer4/16
  Char_COMMA/5(Column_5(1B)) -> 16_to_1_Byte_Multiplexer4/15
  Char_EXCLAMATION_MARK/5(Column_5(1B)) -> 16_to_1_Byte_Multiplexer4/13
  Char_QUESTION_MARK/5(Column_5(1B)) -> 16_to_1_Byte_Multiplexer4/14
  Char_QUOTE/5(Column_5(1B)) -> 16_to_1_Byte_Multiplexer4/12
  Char_SHARP/5(Column_5(1B)) -> 16_to_1_Byte_Multiplexer4/11
  Char_PERCENT/5(Column_5(1B)) -> 16_to_1_Byte_Multiplexer4/10
  Char_LEFT_PARENTHESES/5(Column_5(1B)) -> 16_to_1_Byte_Multiplexer4/9
  Char_RIGHT_PARENTHESES/5(Column_5(1B)) -> 16_to_1_Byte_Multiplexer4/8
  Char_SPACE/5(Column_5(1B)) -> 16_to_1_Byte_Multiplexer4/7
  Char_CURSOR/5(Column_5(1B)) -> 16_to_1_Byte_Multiplexer4/6
  Char_RECTANGLE/5(Column_5(1B)) -> 16_to_1_Byte_Multiplexer4/5
  Char_ARROW_DOWN/6(Column_6(1B)) -> 16_to_1_Byte_Multiplexer5/20
  Char_ARROW_LEFT/6(Column_6(1B)) -> 16_to_1_Byte_Multiplexer5/19
  Char_ARROW_RIGHT/6(Column_6(1B)) -> 16_to_1_Byte_Multiplexer5/18
  Char_UNDERSCORE/6(Column_6(1B)) -> 16_to_1_Byte_Multiplexer5/17
  Char_DOT/6(Column_6(1B)) -> 16_to_1_Byte_Multiplexer5/16
  Char_COMMA/6(Column_6(1B)) -> 16_to_1_Byte_Multiplexer5/15
  Char_QUESTION_MARK/6(Column_6(1B)) -> 16_to_1_Byte_Multiplexer5/14
  Char_EXCLAMATION_MARK/6(Column_6(1B)) -> 16_to_1_Byte_Multiplexer5/13
  Char_QUOTE/6(Column_6(1B)) -> 16_to_1_Byte_Multiplexer5/12
  Char_SHARP/6(Column_6(1B)) -> 16_to_1_Byte_Multiplexer5/11
  Char_PERCENT/6(Column_6(1B)) -> 16_to_1_Byte_Multiplexer5/10
  Char_LEFT_PARENTHESES/6(Column_6(1B)) -> 16_to_1_Byte_Multiplexer5/9
  Char_RIGHT_PARENTHESES/7(Column_7(1B)) -> 16_to_1_Byte_Multiplexer6/8
  Char_RIGHT_PARENTHESES/6(Column_6(1B)) -> 16_to_1_Byte_Multiplexer5/8
  Char_SPACE/6(Column_6(1B)) -> 16_to_1_Byte_Multiplexer5/7
  Char_CURSOR/6(Column_6(1B)) -> 16_to_1_Byte_Multiplexer5/6
  Char_RECTANGLE/6(Column_6(1B)) -> 16_to_1_Byte_Multiplexer5/5
  Char_ARROW_DOWN/7(Column_7(1B)) -> 16_to_1_Byte_Multiplexer6/20
  Char_ARROW_LEFT/7(Column_7(1B)) -> 16_to_1_Byte_Multiplexer6/19
  Char_ARROW_RIGHT/7(Column_7(1B)) -> 16_to_1_Byte_Multiplexer6/18
  Char_UNDERSCORE/7(Column_7(1B)) -> 16_to_1_Byte_Multiplexer6/17
  Char_DOT/7(Column_7(1B)) -> 16_to_1_Byte_Multiplexer6/16
  Char_COMMA/7(Column_7(1B)) -> 16_to_1_Byte_Multiplexer6/15
  Char_QUESTION_MARK/7(Column_7(1B)) -> 16_to_1_Byte_Multiplexer6/14
  Char_EXCLAMATION_MARK/7(Column_7(1B)) -> 16_to_1_Byte_Multiplexer6/13
  Char_QUOTE/7(Column_7(1B)) -> 16_to_1_Byte_Multiplexer6/12
  Char_SHARP/7(Column_7(1B)) -> 16_to_1_Byte_Multiplexer6/11
  Char_PERCENT/7(Column_7(1B)) -> 16_to_1_Byte_Multiplexer6/10
  Char_LEFT_PARENTHESES/7(Column_7(1B)) -> 16_to_1_Byte_Multiplexer6/9
  Char_SPACE/7(Column_7(1B)) -> 16_to_1_Byte_Multiplexer6/7
  Char_CURSOR/7(Column_7(1B)) -> 16_to_1_Byte_Multiplexer6/6
  Char_RECTANGLE/7(Column_7(1B)) -> 16_to_1_Byte_Multiplexer6/5
  Char_ARROW_DOWN/8(Column_8(1B)) -> 16_to_1_Byte_Multiplexer7/20
  Char_ARROW_LEFT/8(Column_8(1B)) -> 16_to_1_Byte_Multiplexer7/19
  Char_ARROW_RIGHT/8(Column_8(1B)) -> 16_to_1_Byte_Multiplexer7/18
  Char_UNDERSCORE/8(Column_8(1B)) -> 16_to_1_Byte_Multiplexer7/17
  Char_DOT/8(Column_8(1B)) -> 16_to_1_Byte_Multiplexer7/16
  Char_COMMA/8(Column_8(1B)) -> 16_to_1_Byte_Multiplexer7/15
  Char_QUESTION_MARK/8(Column_8(1B)) -> 16_to_1_Byte_Multiplexer7/14
  Char_EXCLAMATION_MARK/8(Column_8(1B)) -> 16_to_1_Byte_Multiplexer7/13
  Char_QUOTE/8(Column_8(1B)) -> 16_to_1_Byte_Multiplexer7/12
  Char_SHARP/8(Column_8(1B)) -> 16_to_1_Byte_Multiplexer7/11
  Char_PERCENT/8(Column_8(1B)) -> 16_to_1_Byte_Multiplexer7/10
  Char_LEFT_PARENTHESES/8(Column_8(1B)) -> 16_to_1_Byte_Multiplexer7/9
  Char_RIGHT_PARENTHESES/8(Column_8(1B)) -> 16_to_1_Byte_Multiplexer7/8
  Char_SPACE/8(Column_8(1B)) -> 16_to_1_Byte_Multiplexer7/7
  Char_CURSOR/8(Column_8(1B)) -> 16_to_1_Byte_Multiplexer7/6
  Char_RECTANGLE/8(Column_8(1B)) -> 16_to_1_Byte_Multiplexer7/5
  16_to_1_Byte_Multiplexer/1 -> Column_1(1B)/1
  16_to_1_Byte_Multiplexer1/1 -> Column_2(1B)/1
  16_to_1_Byte_Multiplexer2/1 -> Column_3(1B)/1
  16_to_1_Byte_Multiplexer3/1 -> Column_4(1B)/1
  16_to_1_Byte_Multiplexer4/1 -> Column_5(1B)/1
  16_to_1_Byte_Multiplexer5/1 -> Column_6(1B)/1
  16_to_1_Byte_Multiplexer6/1 -> Column_7(1B)/1
  16_to_1_Byte_Multiplexer7/1 -> Column_8(1B)/1
  Address_0_In(1b)/1 -> 16_to_1_Byte_Multiplexer/4, 16_to_1_Byte_Multiplexer1/4, 16_to_1_Byte_Multiplexer2/4, 16_to_1_Byte_Multiplexer3/4, 16_to_1_Byte_Multiplexer4/4, 16_to_1_Byte_Multiplexer5/4, 16_to_1_Byte_Multiplexer6/4, 16_to_1_Byte_Multiplexer7/4
  Address_1_In(1b)/1 -> 16_to_1_Byte_Multiplexer/3, 16_to_1_Byte_Multiplexer1/3, 16_to_1_Byte_Multiplexer2/3, 16_to_1_Byte_Multiplexer3/3, 16_to_1_Byte_Multiplexer4/3, 16_to_1_Byte_Multiplexer5/3, 16_to_1_Byte_Multiplexer6/3, 16_to_1_Byte_Multiplexer7/3
  Address_2_In(1b)/1 -> 16_to_1_Byte_Multiplexer/2, 16_to_1_Byte_Multiplexer1/2, 16_to_1_Byte_Multiplexer2/2, 16_to_1_Byte_Multiplexer3/2, 16_to_1_Byte_Multiplexer4/2, 16_to_1_Byte_Multiplexer5/2, 16_to_1_Byte_Multiplexer6/2, 16_to_1_Byte_Multiplexer7/2
  Address_3_In(1b)/1 -> 16_to_1_Byte_Multiplexer/1, 16_to_1_Byte_Multiplexer1/1, 16_to_1_Byte_Multiplexer2/1, 16_to_1_Byte_Multiplexer3/1, 16_to_1_Byte_Multiplexer4/1, 16_to_1_Byte_Multiplexer5/1, 16_to_1_Byte_Multiplexer6/1, 16_to_1_Byte_Multiplexer7/1

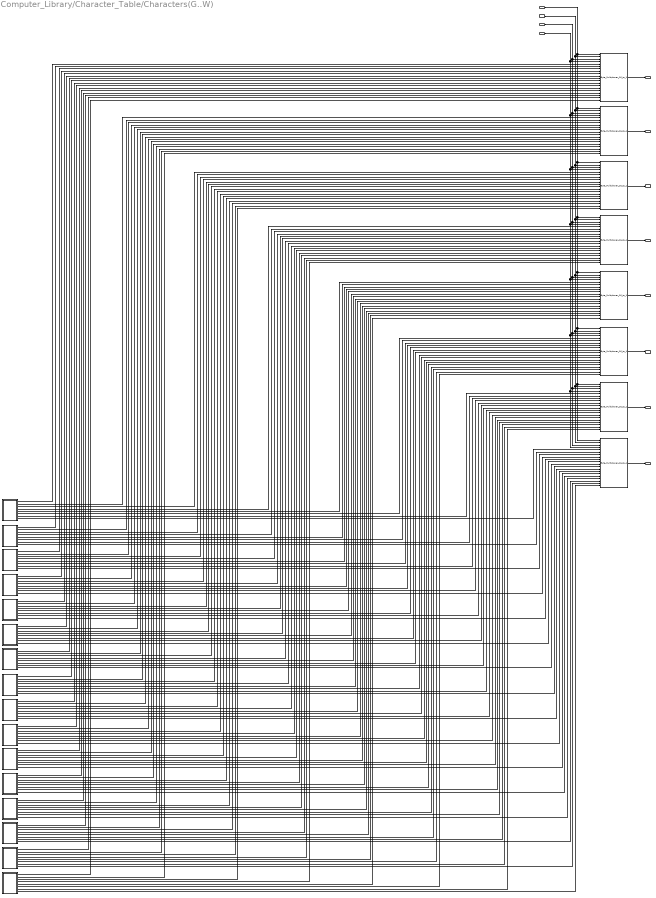
== system Computer_Library/Character_Table/Characters(G..W) ==
  Address_3_In(1b) : Inport
  Address_2_In(1b) : Inport  Port=2
  Address_1_In(1b) : Inport  Port=3
  Address_0_In(1b) : Inport  Port=4
  16_to_1_Byte_Multiplexer{,1..7} (8 alike) : Byte_Multiplexers_Lib/Byte_Multiplexers_Lib/Byte_Multiplexer_16_to_1
  Char_G : Subsystem
  Char_H : Subsystem
  Char_I : Subsystem
  Char_J : Subsystem
  Char_K : Subsystem
  Char_L : Subsystem
  Char_M : Subsystem
  Char_N : Subsystem
  Char_O : Subsystem
  Char_P : Subsystem
  Char_R : Subsystem
  Char_S : Subsystem
  Char_T : Subsystem
  Char_U : Subsystem
  Char_V : Subsystem
  Char_W : Subsystem
  Column_1(1B) : Outport
  Column_2(1B) : Outport  Port=2
  Column_3(1B) : Outport  Port=3
  Column_4(1B) : Outport  Port=4
  Column_5(1B) : Outport  Port=5
  Column_6(1B) : Outport  Port=6
  Column_7(1B) : Outport  Port=7
  Column_8(1B) : Outport  Port=8
  wires:
  Char_W/1(Column_1(1B)) -> 16_to_1_Byte_Multiplexer/5
  Char_V/1(Column_1(1B)) -> 16_to_1_Byte_Multiplexer/6
  Char_U/1(Column_1(1B)) -> 16_to_1_Byte_Multiplexer/7
  Char_T/1(Column_1(1B)) -> 16_to_1_Byte_Multiplexer/8
  Char_S/1(Column_1(1B)) -> 16_to_1_Byte_Multiplexer/9
  Char_R/1(Column_1(1B)) -> 16_to_1_Byte_Multiplexer/10
  Char_P/1(Column_1(1B)) -> 16_to_1_Byte_Multiplexer/11
  Char_O/1(Column_1(1B)) -> 16_to_1_Byte_Multiplexer/12
  Char_N/1(Column_1(1B)) -> 16_to_1_Byte_Multiplexer/13
  Char_M/1(Column_1(1B)) -> 16_to_1_Byte_Multiplexer/14
  Char_L/1(Column_1(1B)) -> 16_to_1_Byte_Multiplexer/15
  Char_K/1(Column_1(1B)) -> 16_to_1_Byte_Multiplexer/16
  Char_J/1(Column_1(1B)) -> 16_to_1_Byte_Multiplexer/17
  Char_I/1(Column_1(1B)) -> 16_to_1_Byte_Multiplexer/18
  Char_H/1(Column_1(1B)) -> 16_to_1_Byte_Multiplexer/19
  Char_G/1(Column_1(1B)) -> 16_to_1_Byte_Multiplexer/20
  Char_W/2(Column_2(1B)) -> 16_to_1_Byte_Multiplexer1/5
  Char_G/2(Column_2(1B)) -> 16_to_1_Byte_Multiplexer1/20
  Char_H/2(Column_2(1B)) -> 16_to_1_Byte_Multiplexer1/19
  Char_I/2(Column_2(1B)) -> 16_to_1_Byte_Multiplexer1/18
  Char_J/2(Column_2(1B)) -> 16_to_1_Byte_Multiplexer1/17
  Char_K/2(Column_2(1B)) -> 16_to_1_Byte_Multiplexer1/16
  Char_L/2(Column_2(1B)) -> 16_to_1_Byte_Multiplexer1/15
  Char_M/2(Column_2(1B)) -> 16_to_1_Byte_Multiplexer1/14
  Char_N/2(Column_2(1B)) -> 16_to_1_Byte_Multiplexer1/13
  Char_O/2(Column_2(1B)) -> 16_to_1_Byte_Multiplexer1/12
  Char_P/2(Column_2(1B)) -> 16_to_1_Byte_Multiplexer1/11
  Char_R/2(Column_2(1B)) -> 16_to_1_Byte_Multiplexer1/10
  Char_S/2(Column_2(1B)) -> 16_to_1_Byte_Multiplexer1/9
  Char_T/2(Column_2(1B)) -> 16_to_1_Byte_Multiplexer1/8
  Char_U/2(Column_2(1B)) -> 16_to_1_Byte_Multiplexer1/7
  Char_V/2(Column_2(1B)) -> 16_to_1_Byte_Multiplexer1/6
  Char_G/3(Column_3(1B)) -> 16_to_1_Byte_Multiplexer2/20
  Char_H/3(Column_3(1B)) -> 16_to_1_Byte_Multiplexer2/19
  Char_I/3(Column_3(1B)) -> 16_to_1_Byte_Multiplexer2/18
  Char_J/3(Column_3(1B)) -> 16_to_1_Byte_Multiplexer2/17
  Char_K/3(Column_3(1B)) -> 16_to_1_Byte_Multiplexer2/16
  Char_L/3(Column_3(1B)) -> 16_to_1_Byte_Multiplexer2/15
  Char_M/3(Column_3(1B)) -> 16_to_1_Byte_Multiplexer2/14
  Char_N/3(Column_3(1B)) -> 16_to_1_Byte_Multiplexer2/13
  Char_O/3(Column_3(1B)) -> 16_to_1_Byte_Multiplexer2/12
  Char_P/3(Column_3(1B)) -> 16_to_1_Byte_Multiplexer2/11
  Char_R/3(Column_3(1B)) -> 16_to_1_Byte_Multiplexer2/10
  Char_S/3(Column_3(1B)) -> 16_to_1_Byte_Multiplexer2/9
  Char_T/3(Column_3(1B)) -> 16_to_1_Byte_Multiplexer2/8
  Char_U/3(Column_3(1B)) -> 16_to_1_Byte_Multiplexer2/7
  Char_V/3(Column_3(1B)) -> 16_to_1_Byte_Multiplexer2/6
  Char_W/3(Column_3(1B)) -> 16_to_1_Byte_Multiplexer2/5
  Char_G/4(Column_4(1B)) -> 16_to_1_Byte_Multiplexer3/20
  Char_H/4(Column_4(1B)) -> 16_to_1_Byte_Multiplexer3/19
  Char_I/4(Column_4(1B)) -> 16_to_1_Byte_Multiplexer3/18
  Char_J/4(Column_4(1B)) -> 16_to_1_Byte_Multiplexer3/17
  Char_K/4(Column_4(1B)) -> 16_to_1_Byte_Multiplexer3/16
  Char_L/4(Column_4(1B)) -> 16_to_1_Byte_Multiplexer3/15
  Char_M/4(Column_4(1B)) -> 16_to_1_Byte_Multiplexer3/14
  Char_N/4(Column_4(1B)) -> 16_to_1_Byte_Multiplexer3/13
  Char_O/4(Column_4(1B)) -> 16_to_1_Byte_Multiplexer3/12
  Char_P/4(Column_4(1B)) -> 16_to_1_Byte_Multiplexer3/11
  Char_R/4(Column_4(1B)) -> 16_to_1_Byte_Multiplexer3/10
  Char_S/4(Column_4(1B)) -> 16_to_1_Byte_Multiplexer3/9
  Char_T/4(Column_4(1B)) -> 16_to_1_Byte_Multiplexer3/8
  Char_U/4(Column_4(1B)) -> 16_to_1_Byte_Multiplexer3/7
  Char_V/4(Column_4(1B)) -> 16_to_1_Byte_Multiplexer3/6
  Char_W/4(Column_4(1B)) -> 16_to_1_Byte_Multiplexer3/5
  Char_G/5(Column_5(1B)) -> 16_to_1_Byte_Multiplexer4/20
  Char_H/5(Column_5(1B)) -> 16_to_1_Byte_Multiplexer4/19
  Char_I/5(Column_5(1B)) -> 16_to_1_Byte_Multiplexer4/18
  Char_J/5(Column_5(1B)) -> 16_to_1_Byte_Multiplexer4/17
  Char_K/5(Column_5(1B)) -> 16_to_1_Byte_Multiplexer4/16
  Char_L/5(Column_5(1B)) -> 16_to_1_Byte_Multiplexer4/15
  Char_N/5(Column_5(1B)) -> 16_to_1_Byte_Multiplexer4/13
  Char_M/5(Column_5(1B)) -> 16_to_1_Byte_Multiplexer4/14
  Char_O/5(Column_5(1B)) -> 16_to_1_Byte_Multiplexer4/12
  Char_P/5(Column_5(1B)) -> 16_to_1_Byte_Multiplexer4/11
  Char_R/5(Column_5(1B)) -> 16_to_1_Byte_Multiplexer4/10
  Char_S/5(Column_5(1B)) -> 16_to_1_Byte_Multiplexer4/9
  Char_T/5(Column_5(1B)) -> 16_to_1_Byte_Multiplexer4/8
  Char_U/5(Column_5(1B)) -> 16_to_1_Byte_Multiplexer4/7
  Char_V/5(Column_5(1B)) -> 16_to_1_Byte_Multiplexer4/6
  Char_W/5(Column_5(1B)) -> 16_to_1_Byte_Multiplexer4/5
  Char_G/6(Column_6(1B)) -> 16_to_1_Byte_Multiplexer5/20
  Char_H/6(Column_6(1B)) -> 16_to_1_Byte_Multiplexer5/19
  Char_I/6(Column_6(1B)) -> 16_to_1_Byte_Multiplexer5/18
  Char_J/6(Column_6(1B)) -> 16_to_1_Byte_Multiplexer5/17
  Char_K/6(Column_6(1B)) -> 16_to_1_Byte_Multiplexer5/16
  Char_L/6(Column_6(1B)) -> 16_to_1_Byte_Multiplexer5/15
  Char_M/6(Column_6(1B)) -> 16_to_1_Byte_Multiplexer5/14
  Char_N/6(Column_6(1B)) -> 16_to_1_Byte_Multiplexer5/13
  Char_O/6(Column_6(1B)) -> 16_to_1_Byte_Multiplexer5/12
  Char_P/6(Column_6(1B)) -> 16_to_1_Byte_Multiplexer5/11
  Char_R/6(Column_6(1B)) -> 16_to_1_Byte_Multiplexer5/10
  Char_S/6(Column_6(1B)) -> 16_to_1_Byte_Multiplexer5/9
  Char_T/7(Column_7(1B)) -> 16_to_1_Byte_Multiplexer6/8
  Char_T/6(Column_6(1B)) -> 16_to_1_Byte_Multiplexer5/8
  Char_U/6(Column_6(1B)) -> 16_to_1_Byte_Multiplexer5/7
  Char_V/6(Column_6(1B)) -> 16_to_1_Byte_Multiplexer5/6
  Char_W/6(Column_6(1B)) -> 16_to_1_Byte_Multiplexer5/5
  Char_G/7(Column_7(1B)) -> 16_to_1_Byte_Multiplexer6/20
  Char_H/7(Column_7(1B)) -> 16_to_1_Byte_Multiplexer6/19
  Char_I/7(Column_7(1B)) -> 16_to_1_Byte_Multiplexer6/18
  Char_J/7(Column_7(1B)) -> 16_to_1_Byte_Multiplexer6/17
  Char_K/7(Column_7(1B)) -> 16_to_1_Byte_Multiplexer6/16
  Char_L/7(Column_7(1B)) -> 16_to_1_Byte_Multiplexer6/15
  Char_M/7(Column_7(1B)) -> 16_to_1_Byte_Multiplexer6/14
  Char_N/7(Column_7(1B)) -> 16_to_1_Byte_Multiplexer6/13
  Char_O/7(Column_7(1B)) -> 16_to_1_Byte_Multiplexer6/12
  Char_P/7(Column_7(1B)) -> 16_to_1_Byte_Multiplexer6/11
  Char_R/7(Column_7(1B)) -> 16_to_1_Byte_Multiplexer6/10
  Char_S/7(Column_7(1B)) -> 16_to_1_Byte_Multiplexer6/9
  Char_U/7(Column_7(1B)) -> 16_to_1_Byte_Multiplexer6/7
  Char_V/7(Column_7(1B)) -> 16_to_1_Byte_Multiplexer6/6
  Char_W/7(Column_7(1B)) -> 16_to_1_Byte_Multiplexer6/5
  Char_G/8(Column_8(1B)) -> 16_to_1_Byte_Multiplexer7/20
  Char_H/8(Column_8(1B)) -> 16_to_1_Byte_Multiplexer7/19
  Char_I/8(Column_8(1B)) -> 16_to_1_Byte_Multiplexer7/18
  Char_J/8(Column_8(1B)) -> 16_to_1_Byte_Multiplexer7/17
  Char_K/8(Column_8(1B)) -> 16_to_1_Byte_Multiplexer7/16
  Char_L/8(Column_8(1B)) -> 16_to_1_Byte_Multiplexer7/15
  Char_M/8(Column_8(1B)) -> 16_to_1_Byte_Multiplexer7/14
  Char_N/8(Column_8(1B)) -> 16_to_1_Byte_Multiplexer7/13
  Char_O/8(Column_8(1B)) -> 16_to_1_Byte_Multiplexer7/12
  Char_P/8(Column_8(1B)) -> 16_to_1_Byte_Multiplexer7/11
  Char_R/8(Column_8(1B)) -> 16_to_1_Byte_Multiplexer7/10
  Char_S/8(Column_8(1B)) -> 16_to_1_Byte_Multiplexer7/9
  Char_T/8(Column_8(1B)) -> 16_to_1_Byte_Multiplexer7/8
  Char_U/8(Column_8(1B)) -> 16_to_1_Byte_Multiplexer7/7
  Char_V/8(Column_8(1B)) -> 16_to_1_Byte_Multiplexer7/6
  Char_W/8(Column_8(1B)) -> 16_to_1_Byte_Multiplexer7/5
  16_to_1_Byte_Multiplexer/1 -> Column_1(1B)/1
  16_to_1_Byte_Multiplexer1/1 -> Column_2(1B)/1
  16_to_1_Byte_Multiplexer2/1 -> Column_3(1B)/1
  16_to_1_Byte_Multiplexer3/1 -> Column_4(1B)/1
  16_to_1_Byte_Multiplexer4/1 -> Column_5(1B)/1
  16_to_1_Byte_Multiplexer5/1 -> Column_6(1B)/1
  16_to_1_Byte_Multiplexer6/1 -> Column_7(1B)/1
  16_to_1_Byte_Multiplexer7/1 -> Column_8(1B)/1
  Address_0_In(1b)/1 -> 16_to_1_Byte_Multiplexer/4, 16_to_1_Byte_Multiplexer1/4, 16_to_1_Byte_Multiplexer2/4, 16_to_1_Byte_Multiplexer3/4, 16_to_1_Byte_Multiplexer4/4, 16_to_1_Byte_Multiplexer5/4, 16_to_1_Byte_Multiplexer6/4, 16_to_1_Byte_Multiplexer7/4
  Address_1_In(1b)/1 -> 16_to_1_Byte_Multiplexer/3, 16_to_1_Byte_Multiplexer1/3, 16_to_1_Byte_Multiplexer2/3, 16_to_1_Byte_Multiplexer3/3, 16_to_1_Byte_Multiplexer4/3, 16_to_1_Byte_Multiplexer5/3, 16_to_1_Byte_Multiplexer6/3, 16_to_1_Byte_Multiplexer7/3
  Address_2_In(1b)/1 -> 16_to_1_Byte_Multiplexer/2, 16_to_1_Byte_Multiplexer1/2, 16_to_1_Byte_Multiplexer2/2, 16_to_1_Byte_Multiplexer3/2, 16_to_1_Byte_Multiplexer4/2, 16_to_1_Byte_Multiplexer5/2, 16_to_1_Byte_Multiplexer6/2, 16_to_1_Byte_Multiplexer7/2
  Address_3_In(1b)/1 -> 16_to_1_Byte_Multiplexer/1, 16_to_1_Byte_Multiplexer1/1, 16_to_1_Byte_Multiplexer2/1, 16_to_1_Byte_Multiplexer3/1, 16_to_1_Byte_Multiplexer4/1, 16_to_1_Byte_Multiplexer5/1, 16_to_1_Byte_Multiplexer6/1, 16_to_1_Byte_Multiplexer7/1
